simulink model "default"  (R2024b)
settings: Solver=VariableStepAuto  StartTime=0.0  StopTime=10.0  RelTol=1e-3
settings Model: Creator=Koupanis  LastModifiedBy=Koupanis

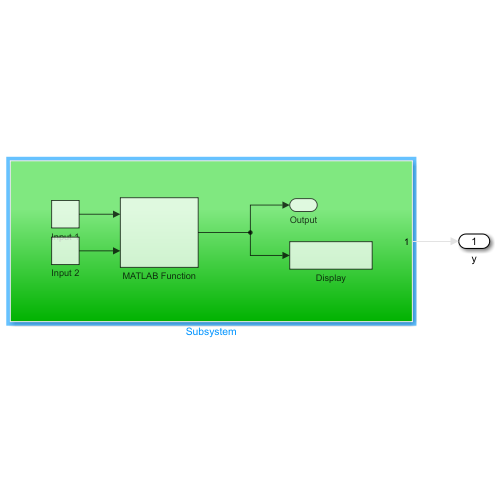
[thumbnail: Simulink's stored preview of the top-level diagram]
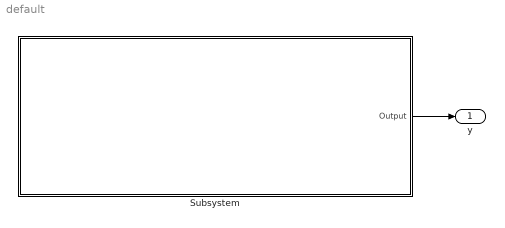
== system default ==
  Subsystem : Subsystem
  y : Outport
  wires:
  Subsystem/1(Output) -> y/1

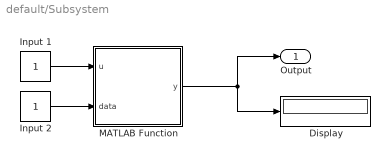
== system default/Subsystem ==
  Display : Display
  Input 1 : Constant
  Input 2 : Constant
  MATLAB Function : MATLAB Function  TreatAsAtomicUnit=on
  Output : Outport
  wires:
  Input 2/1 -> MATLAB Function/2(data)
  MATLAB Function/1(y) -> Output/1, Display/1
  Input 1/1 -> MATLAB Function/1(u)

== matlab function default/Subsystem/MATLAB Function ==
  data: u input; y output; data input
function y = fcn(u, data)

y = u;
